simulink model "ten_to_64"  (R2012b)
settings: Solver=FixedStepDiscrete  SolverMode=SingleTasking  StartTime=0.0  StopTime=20000  FixedStep=1  RelTol=1e-3
libraries: xbsIndex_r4 x424, xps_library x1
(part 1 of 3)
settings Model: Creator=paulp  LastModifiedBy=paulp
settings DataIOCC: LimitDataPoints=off
settings OptimizationCC: SimCompilerOptimization=On

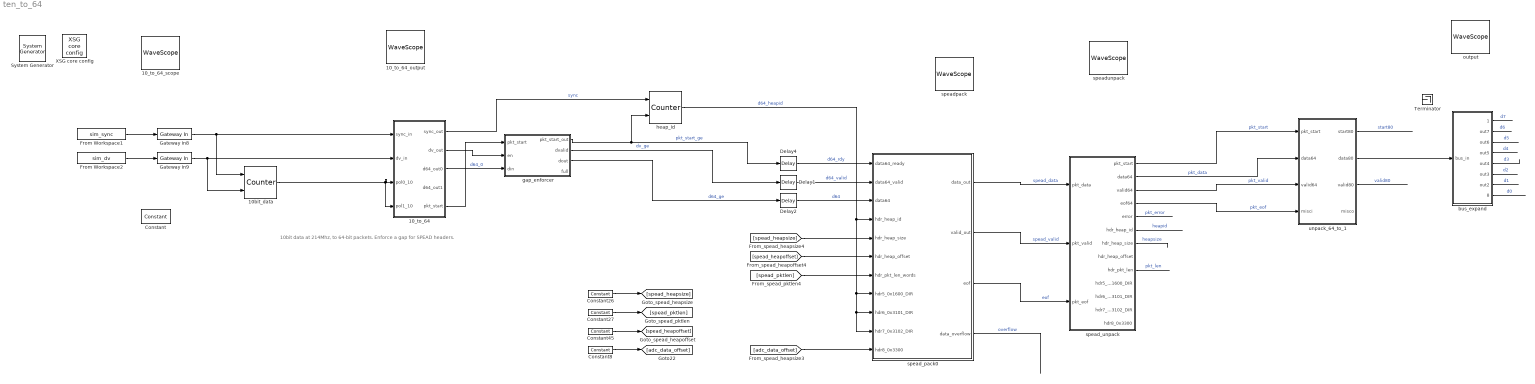
== system ten_to_64 ==
  note: 10bit data at 214Mhz, to 64-bit packets.
      | Enforce a gap for SPEAD headers.
  " System Generator" : xbsIndex_r4/ System Generator  Tag=genX  xilinxfamily=virtex6  part=xc6vsx475t  speed=-1  package=ff1759  synthesis_tool=XST  clock_wrapper=Clock Enables  directory=./netlist  proj_type=Project Navigator  Synth_file=XST Defaults  Impl_file=ISE Defaults  testbench=off  simulink_period=1  sysclk_period=10  dcm_input_clock_period=10  incr_netlist=off  trim_vbits=Everywhere in SubSystem  dbl_ovrd=According to Block Masks  core_generation=According to Block Masks  run_coregen=off  deprecated_control=off  eval_field=0  block_type=sysgen
  10_to_64 : Subsystem
  10_to_64_output : xbsIndex_r4/WaveScope  block_type=wavescope
  10_to_64_scope : xbsIndex_r4/WaveScope  block_type=wavescope
  10bit_data : xbsIndex_r4/Counter  cnt_type=Free Running  cnt_to=Inf  operation=Up  start_count=0  cnt_by_val=1  arith_type=Unsigned  n_bits=10  bin_pt=0  load_pin=off  rst=on  en=on  explicit_period=on  period=1  dbl_ovrd=off  use_behavioral_HDL=off  implementation=Fabric  block_type=counter
  Constant : xbsIndex_r4/Constant  const=1  gui_display_data_type=Boolean  arith_type=Boolean  n_bits=16  bin_pt=14  preci_type=Single  exp_width=8  frac_width=24  explicit_period=on  period=1  equ=P=C  opselect=C  inp2=PCIN>>17  opr=+  inp1=P  carry=CIN  dbl_ovrd=off  block_type=constant
  Constant26 : xbsIndex_r4/Constant  const=4096*10/8  gui_display_data_type=Fixed-point  arith_type=Unsigned  n_bits=48  bin_pt=0  preci_type=Single  exp_width=8  frac_width=24  explicit_period=on  period=1  equ=P=C  opselect=C  inp2=PCIN>>17  opr=+  inp1=P  carry=CIN  dbl_ovrd=off  block_type=constant
  Constant27 : xbsIndex_r4/Constant  const=(4096*10/8)/8  gui_display_data_type=Fixed-point  arith_type=Unsigned  n_bits=48  bin_pt=0  preci_type=Single  exp_width=8  frac_width=24  explicit_period=on  period=1  equ=P=C  opselect=C  inp2=PCIN>>17  opr=+  inp1=P  carry=CIN  dbl_ovrd=off  block_type=constant
  Constant45 : xbsIndex_r4/Constant  const=0  gui_display_data_type=Fixed-point  arith_type=Unsigned  n_bits=48  bin_pt=0  preci_type=Single  exp_width=8  frac_width=24  explicit_period=on  period=1  equ=P=C  opselect=C  inp2=PCIN>>17  opr=+  inp1=P  carry=CIN  dbl_ovrd=off  block_type=constant
  Constant8 : xbsIndex_r4/Constant  const=0  gui_display_data_type=Fixed-point  arith_type=Unsigned  n_bits=48  bin_pt=0  preci_type=Single  exp_width=8  frac_width=24  explicit_period=on  period=1  equ=P=C  opselect=C  inp2=PCIN>>17  opr=+  inp1=P  carry=CIN  dbl_ovrd=off  block_type=constant
  Delay1 : xbsIndex_r4/Delay  rst=off  infoeditControl=Selection of Reset will increase slice count due to use of real FFs and instead of SRLs  en=off  latency=1  dbl_ovrd=off  reg_retiming=off  block_type=delay
  Delay2 : xbsIndex_r4/Delay  rst=off  infoeditControl=Selection of Reset will increase slice count due to use of real FFs and instead of SRLs  en=off  latency=1  dbl_ovrd=off  reg_retiming=off  block_type=delay
  Delay4 : xbsIndex_r4/Delay  rst=off  infoeditControl=Selection of Reset will increase slice count due to use of real FFs and instead of SRLs  en=off  latency=1  dbl_ovrd=off  reg_retiming=off  block_type=delay
  From Workspace1 : FromWorkspace  VariableName=sim_sync  SampleTime=1  Interpolate=off  OutputAfterFinalValue=Setting to zero
  From Workspace2 : FromWorkspace  VariableName=sim_dv  SampleTime=1  Interpolate=off  OutputAfterFinalValue=Setting to zero
  Gateway In8 : xbsIndex_r4/Gateway In  gui_display_data_type=Boolean  arith_type=Boolean  n_bits=10  bin_pt=9  preci_type=Single  exp_width=8  frac_width=24  quantization="Round  (unbiased: +/- Inf)"  overflow=Saturate  period=1  dbl_ovrd=off  timing_constraint=None  locs_specified=off  LOCs={}  UseAsADC=off  ADCChannel='1'  inherit_from_input=off  hdl_port=on  block_type=gatewayin
  Gateway In9 : xbsIndex_r4/Gateway In  gui_display_data_type=Boolean  arith_type=Boolean  n_bits=10  bin_pt=9  preci_type=Single  exp_width=8  frac_width=24  quantization="Round  (unbiased: +/- Inf)"  overflow=Saturate  period=1  dbl_ovrd=off  timing_constraint=None  locs_specified=off  LOCs={}  UseAsADC=off  ADCChannel='1'  inherit_from_input=off  hdl_port=on  block_type=gatewayin
  Terminator : Terminator
  XSG core config : xps_library/XSG core config  Tag=xps:xsg  hw_sys=ROACH2:sx475t  clk_src=sys_clk  ROACH_clk_src=sys_clk  ROACH2_clk_src=sys_clk  MKDIG_clk_src=sys_clk  clk_rate=229  sample_period=1  synthesis_tool=XST
  bus_expand : Subsystem  AncestorBlock=casper_library_flow_control/bus_expand  mask(bus_expand){mode=divisions of equal size, outputNum=8, outputWidth=10, outputBinaryPt=0, outputArithmeticType=0, show_format=on, outputToWorkspace=off, variablePrefix=out, outputToModelAsWell=on}
      mask prompts: outputNum "Number of outputs:"; outputWidth "Output width:"; outputBinaryPt "Output binary point position:"; outputArithmeticType "Output arithmetic type (ufix=0, fix=1, bool=2):"; show_format "Print format string?"; outputToWorkspace "Output to workspace?"; variablePrefix "Variable name prefix:"; outputToModelAsWell "Output to model as well?"
      mask help:
      | Expands a 'bus' made using a bus_create or Xilinx
      | concat block.
      | The input will be divided into the specified number
      | of outputs with the specified arithmetic types.
      | Divisions are made from most significant bit.
      mask init:
      | bus_expand_init(gcb,...
      |     'mode', mode, ...
      |     'outputNum', outputNum, ...
      |     'outputWidth', outputWidth, ...
      |     'outputBinaryPt', outputBinaryPt, ...
      |     'outputArithmeticType', outputArithmeticType, ...
      |     'show_format', show_format, ...
      |     'outputToWorkspace', outputToWorkspace, ...
      |     'variablePrefix', variablePrefix, ...
      |     'outputToModelAsWell', outputToModelAsWell);
      settings: AttributesFormatString=8 outputs: uf10.0,uf10.0,uf10.0,uf10.0,uf10.0,uf10.0,uf10.0,uf10.0,
      mask TypeOptions mode: divisions of equal size | divisions of arbitrary size
      mask Callback mode: bus_expand_callback();
      mask Callback outputWidth: bus_expand_callback();
      mask Callback outputToWorkspace: bus_expand_callback();
  gap_enforcer : Subsystem  mask{block_size=2^(8-1), gap_size=15}
      mask prompts: block_size "data block size"; gap_size "gap size"
  heap_id : xbsIndex_r4/Counter  cnt_type=Free Running  cnt_to=Inf  operation=Up  start_count=0  cnt_by_val=1  arith_type=Unsigned  n_bits=48  bin_pt=0  load_pin=off  rst=on  en=on  explicit_period=on  period=1  dbl_ovrd=off  use_behavioral_HDL=off  implementation=Fabric  block_type=counter
  output : xbsIndex_r4/WaveScope  block_type=wavescope
  spead_pack0 : Subsystem  Tag=casper:spead_pack  AncestorBlock=casper_library_communications/spead_pack  mask(pkt_pack_mask){max_pkt_len_bits=10, header_ids=0x1600, 0x3101, 0x3102, header_ind_ids=0x3300, spead_msw=64, spead_lsw=48, spead_version=4, bytes_per_word=8}
      mask prompts: max_pkt_len_bits "Max pkt length, 2^? 64-bit words"; header_ids "SPEAD direct address IDs (decimal)"; header_ind_ids "SPEAD indirect address IDs (decimal)"; spead_msw "SPEAD Flavour (MSw)"; spead_lsw "SPEAD Flavour (LSw)"; spead_version "SPEAD version"; bytes_per_word "Word size, in bytes"
      mask help:
      | This block generates SPEAD-compliant packets from a datastream.
      |
      | Packets are created with a fixed header followed by a number of 64-bit items.
      |
      | Requires a 64-bit data stream.
      |
      | The data_ready signal is one cycle BEFORE valid data! Does not have to be with a valid signal either.
      mask init:
      | if floor(log2(bytes_per_word)) ~= log2(bytes_per_word)
      |     error('Bytes per word should be a power of two.');
      | end
      | 
      | spead_pack_init(gcb)
  spead_unpack : Subsystem  Tag=casper:spead_unpack  AncestorBlock=casper_library_communications/spead_unpack  mask(spead_unpack_mask){max_pkt_len_bits=10, header_ids=0x1600, 0x3101, 0x3102, header_ind_ids=0x3300, spead_msw=64, spead_lsw=48, spead_version=4, combine_errors=on}
      mask prompts: max_pkt_len_bits "Max pkt length, 2^? 64-bit words"; header_ids "SPEAD direct header IDs (decimal)"; header_ind_ids "SPEAD indirect address IDs (decimal)"; spead_msw "SPEAD Flavour (MSw)"; spead_lsw "SPEAD Flavour (LSw)"; spead_version "SPEAD version"; combine_errors "Combine error flags"
      mask help: This block receives a 64-bit-word stream that contains a SPEAD stream. It checks the SPEAD headers are being correctly received. It presents the user with all headers on the first valid cycle of data along with a flag to indicate a header or packet-length error.
      mask init:
      | spead_unpack_init(gcb)
  speadpack : xbsIndex_r4/WaveScope  block_type=wavescope
  speadunpack : xbsIndex_r4/WaveScope  block_type=wavescope
  unpack_64_to_1 : Subsystem
  wires:
  From Workspace1/1 -> Gateway In8/1
  From Workspace2/1 -> Gateway In9/1
  Gateway In8/1 -> 10bit_data/1, 10_to_64/1(sync_in)
  10bit_data/1 -> 10_to_64/3(pol0_10), 10_to_64/4(pol1_10)
  Gateway In9/1 -> 10bit_data/2, 10_to_64/2(dv_in)
  unpack_64_to_1/1(start80) -> ?  "start80"
  unpack_64_to_1/3(valid80) -> ?  "valid80"
  unpack_64_to_1/2(data80) -> bus_expand/1(bus_in)
  bus_expand/1(msb_out8) -> ?  "d7"
  bus_expand/2(out7) -> ?  "d6"
  bus_expand/3(out6) -> ?  "d5"
  bus_expand/4(out5) -> ?  "d4"
  bus_expand/5(out4) -> ?  "d3"
  bus_expand/6(out3) -> ?  "d2"
  bus_expand/7(out2) -> ?  "d1"
  bus_expand/8(lsb_out1) -> ?  "d0"
  Constant26/1 -> [spead_heapsize]
  Constant27/1 -> [spead_pktlen]
  Constant45/1 -> [spead_heapoffset]
  Constant8/1 -> [adc_data_offset]
  [spead_heapsize] -> spead_pack0/5(hdr_heap_size)
  [spead_heapoffset] -> spead_pack0/6(hdr_heap_offset)
  [spead_pktlen] -> spead_pack0/7(hdr_pkt_len_words)
  [adc_data_offset] -> spead_pack0/11(hdr8_0x3300)
  heap_id/1 -> spead_pack0/10(hdr7_0x3102_DIR), spead_pack0/9(hdr6_0x3101_DIR), spead_pack0/8(hdr5_0x1600_DIR), spead_pack0/4(hdr_heap_id)  "d64_heapid"
  spead_pack0/1(data_out) -> spead_unpack/1(pkt_data)  "spead_data"
  spead_pack0/2(valid_out) -> spead_unpack/2(pkt_valid)  "spead_valid"
  spead_pack0/3(eof) -> spead_unpack/3(pkt_eof)  "eof"
  spead_pack0/4(data_overflow) -> ?  "overflow"
  10_to_64/1(sync_out) -> heap_id/1  "sync"
  10_to_64/3(d64_out0) -> gap_enforcer/3(din)  "d64_0"
  10_to_64/2(dv_out) -> gap_enforcer/2(en)
  spead_unpack/4(eof64) -> unpack_64_to_1/4(misci)  "pkt_eof"
  spead_unpack/6(hdr_heap_id) -> ?  "heapid"
  spead_unpack/5(error) -> ?  "pkt_error"
  spead_unpack/7(hdr_heap_size) -> ?  "heapsize"
  spead_unpack/9(hdr_pkt_len) -> ?  "pkt_len"
  10_to_64/5(pkt_start) -> gap_enforcer/1(pkt_start)
  spead_unpack/1(pkt_start) -> unpack_64_to_1/1(pkt_start)  "pkt_start"
  spead_unpack/2(data64) -> unpack_64_to_1/2(data64)  "pkt_data"
  spead_unpack/3(valid64) -> unpack_64_to_1/3(valid64)  "pkt_valid"
  Delay4/1 -> spead_pack0/1(data64_ready)  "d64_rdy"
  Delay1/1 -> spead_pack0/2(data64_valid)  "d64_valid"
  Delay2/1 -> spead_pack0/3(data64)  "d64"
  gap_enforcer/1(pkt_start_out) -> heap_id/2, Delay4/1  "pkt_start_ge"
  gap_enforcer/2(dvalid) -> Delay1/1  "dv_ge"
  gap_enforcer/3(dout) -> Delay2/1  "d64_ge"

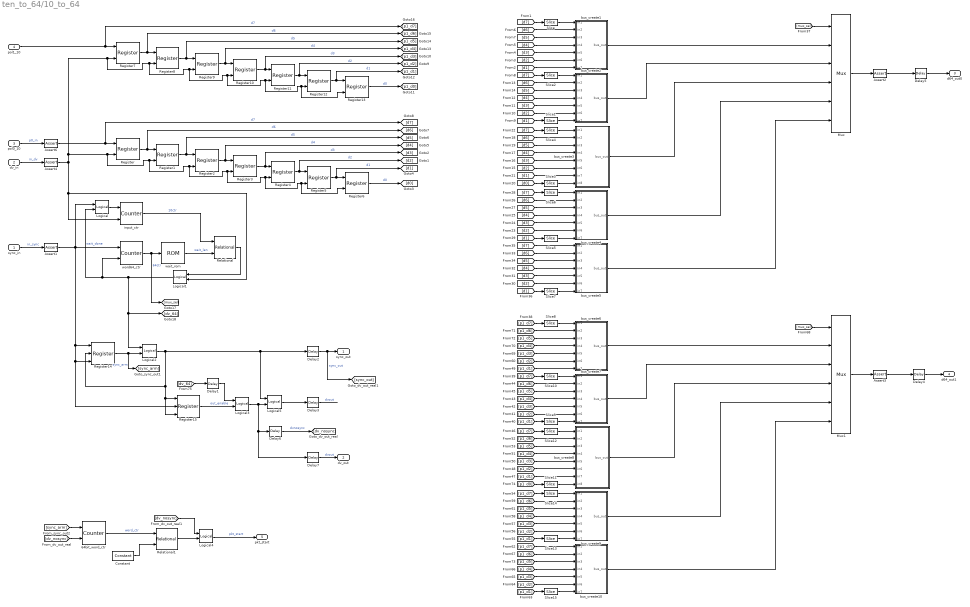
== system ten_to_64/10_to_64 ==
  sync_in : Inport
  dv_in : Inport  Port=2
  pol0_10 : Inport  Port=3
  pol1_10 : Inport  Port=4
  64bit_word_ctr : xbsIndex_r4/Counter  cnt_type=Count Limited  cnt_to=639  operation=Up  start_count=0  cnt_by_val=1  arith_type=Unsigned  n_bits=10  bin_pt=0  load_pin=off  rst=on  en=on  explicit_period=on  period=1  dbl_ovrd=off  use_behavioral_HDL=off  implementation=Fabric  block_type=counter
  Assert1 : xbsIndex_r4/Assert  assert_type=on  type_source=Explicitly  gui_display_data_type=Boolean  arith_type=Boolean  n_bits=80  bin_pt=0  preci_type=Single  exp_width=8  frac_width=24  assert_rate=off  rate_source=Explicitly  period=1  output_port=on  block_type=assert
      settings: block_version=10.1.3
  Assert2 : xbsIndex_r4/Assert  assert_type=on  type_source=Explicitly  gui_display_data_type=Fixed-point  arith_type=Unsigned  n_bits=64  bin_pt=0  preci_type=Single  exp_width=8  frac_width=24  assert_rate=off  rate_source=Explicitly  period=1  output_port=on  block_type=assert
      settings: block_version=10.1.3
  Assert3 : xbsIndex_r4/Assert  assert_type=on  type_source=Explicitly  gui_display_data_type=Fixed-point  arith_type=Unsigned  n_bits=64  bin_pt=0  preci_type=Single  exp_width=8  frac_width=24  assert_rate=off  rate_source=Explicitly  period=1  output_port=on  block_type=assert
      settings: block_version=10.1.3
  Assert4 : xbsIndex_r4/Assert  assert_type=on  type_source=Explicitly  gui_display_data_type=Boolean  arith_type=Boolean  n_bits=80  bin_pt=0  preci_type=Single  exp_width=8  frac_width=24  assert_rate=off  rate_source=Explicitly  period=1  output_port=on  block_type=assert
      settings: block_version=10.1.3
  Assert6 : xbsIndex_r4/Assert  assert_type=on  type_source=Explicitly  gui_display_data_type=Fixed-point  arith_type=Unsigned  n_bits=10  bin_pt=0  preci_type=Single  exp_width=8  frac_width=24  assert_rate=off  rate_source=Explicitly  period=1  output_port=on  block_type=assert
      settings: block_version=10.1.3
  Constant : xbsIndex_r4/Constant  const=0  gui_display_data_type=Fixed-point  arith_type=Unsigned  n_bits=10  bin_pt=0  preci_type=Single  exp_width=8  frac_width=24  explicit_period=on  period=1  equ=P=C  opselect=C  inp2=PCIN>>17  opr=+  inp1=P  carry=CIN  dbl_ovrd=off  block_type=constant
  Delay1 : xbsIndex_r4/Delay  rst=off  infoeditControl=Selection of Reset will increase slice count due to use of real FFs and instead of SRLs  en=off  latency=1  dbl_ovrd=off  reg_retiming=off  block_type=delay
  Delay{2..5,7} (5 alike) : xbsIndex_r4/Delay  rst=off  infoeditControl=Selection of Reset will increase slice count due to use of real FFs and instead of SRLs  en=off  latency=2  dbl_ovrd=off  reg_retiming=off  block_type=delay
  Delay6 : xbsIndex_r4/Delay  rst=off  infoeditControl=Selection of Reset will increase slice count due to use of real FFs and instead of SRLs  en=off  latency=1  dbl_ovrd=off  reg_retiming=off  block_type=delay
  Logical : xbsIndex_r4/Logical  logical_function=OR  inputs=2  en=off  latency=0  precision=Full  arith_type=Unsigned  n_bits=16  bin_pt=0  align_bp=on  dbl_ovrd=off  block_type=logical
  Logical{1..4} (4 alike) : xbsIndex_r4/Logical  logical_function=AND  inputs=2  en=off  latency=0  precision=Full  arith_type=Unsigned  n_bits=16  bin_pt=0  align_bp=on  dbl_ovrd=off  block_type=logical
  Logical5 : xbsIndex_r4/Logical  logical_function=OR  inputs=2  en=off  latency=0  precision=Full  arith_type=Unsigned  n_bits=16  bin_pt=0  align_bp=on  dbl_ovrd=off  block_type=logical
  Mux : xbsIndex_r4/Mux  inputs=5  en=off  latency=1  precision=Full  arith_type=Unsigned  n_bits=16  bin_pt=14  quantization=Truncate  overflow=Wrap  dbl_ovrd=off  block_type=mux
  Mux1 : xbsIndex_r4/Mux  inputs=5  en=off  latency=1  precision=Full  arith_type=Unsigned  n_bits=16  bin_pt=14  quantization=Truncate  overflow=Wrap  dbl_ovrd=off  block_type=mux
  Register{,1..13} (14 alike) : xbsIndex_r4/Register  init=0  rst=off  en=on  dbl_ovrd=off  block_type=register
  Register14 : xbsIndex_r4/Register  init=0  rst=on  en=on  dbl_ovrd=off  block_type=register
  Register15 : xbsIndex_r4/Register  init=0  rst=on  en=on  dbl_ovrd=off  block_type=register
  Relational : xbsIndex_r4/Relational  mode=a=b  en=off  latency=0  dbl_ovrd=off  block_type=relational
  Relational1 : xbsIndex_r4/Relational  mode=a=b  en=off  latency=0  dbl_ovrd=off  block_type=relational
  Slice : xbsIndex_r4/Slice  nbits=4  boolean_output=off  mode=Lower Bit Location + Width  bit1=0  base1=MSB of Input  bit0=0  base0=LSB of Input  dbl_ovrd=off  block_type=slice
  Slice1 : xbsIndex_r4/Slice  nbits=6  boolean_output=off  mode=Upper Bit Location + Width  bit1=0  base1=MSB of Input  bit0=0  base0=LSB of Input  dbl_ovrd=off  block_type=slice
  Slice10 : xbsIndex_r4/Slice  nbits=8  boolean_output=off  mode=Lower Bit Location + Width  bit1=0  base1=MSB of Input  bit0=0  base0=LSB of Input  dbl_ovrd=off  block_type=slice
  Slice11 : xbsIndex_r4/Slice  nbits=2  boolean_output=off  mode=Upper Bit Location + Width  bit1=0  base1=MSB of Input  bit0=0  base0=LSB of Input  dbl_ovrd=off  block_type=slice
  Slice12 : xbsIndex_r4/Slice  nbits=2  boolean_output=off  mode=Lower Bit Location + Width  bit1=0  base1=MSB of Input  bit0=0  base0=LSB of Input  dbl_ovrd=off  block_type=slice
  Slice13 : xbsIndex_r4/Slice  nbits=8  boolean_output=off  mode=Upper Bit Location + Width  bit1=0  base1=MSB of Input  bit0=0  base0=LSB of Input  dbl_ovrd=off  block_type=slice
  Slice14 : xbsIndex_r4/Slice  nbits=6  boolean_output=off  mode=Lower Bit Location + Width  bit1=0  base1=MSB of Input  bit0=0  base0=LSB of Input  dbl_ovrd=off  block_type=slice
  Slice15 : xbsIndex_r4/Slice  nbits=4  boolean_output=off  mode=Upper Bit Location + Width  bit1=0  base1=MSB of Input  bit0=0  base0=LSB of Input  dbl_ovrd=off  block_type=slice
  Slice2 : xbsIndex_r4/Slice  nbits=8  boolean_output=off  mode=Lower Bit Location + Width  bit1=0  base1=MSB of Input  bit0=0  base0=LSB of Input  dbl_ovrd=off  block_type=slice
  Slice3 : xbsIndex_r4/Slice  nbits=2  boolean_output=off  mode=Upper Bit Location + Width  bit1=0  base1=MSB of Input  bit0=0  base0=LSB of Input  dbl_ovrd=off  block_type=slice
  Slice4 : xbsIndex_r4/Slice  nbits=2  boolean_output=off  mode=Lower Bit Location + Width  bit1=0  base1=MSB of Input  bit0=0  base0=LSB of Input  dbl_ovrd=off  block_type=slice
  Slice5 : xbsIndex_r4/Slice  nbits=8  boolean_output=off  mode=Upper Bit Location + Width  bit1=0  base1=MSB of Input  bit0=0  base0=LSB of Input  dbl_ovrd=off  block_type=slice
  Slice6 : xbsIndex_r4/Slice  nbits=6  boolean_output=off  mode=Lower Bit Location + Width  bit1=0  base1=MSB of Input  bit0=0  base0=LSB of Input  dbl_ovrd=off  block_type=slice
  Slice7 : xbsIndex_r4/Slice  nbits=4  boolean_output=off  mode=Upper Bit Location + Width  bit1=0  base1=MSB of Input  bit0=0  base0=LSB of Input  dbl_ovrd=off  block_type=slice
  Slice8 : xbsIndex_r4/Slice  nbits=4  boolean_output=off  mode=Lower Bit Location + Width  bit1=0  base1=MSB of Input  bit0=0  base0=LSB of Input  dbl_ovrd=off  block_type=slice
  Slice9 : xbsIndex_r4/Slice  nbits=6  boolean_output=off  mode=Upper Bit Location + Width  bit1=0  base1=MSB of Input  bit0=0  base0=LSB of Input  dbl_ovrd=off  block_type=slice
  bus_create1 : Subsystem  AncestorBlock=casper_library_flow_control/bus_create  mask(bus_create){inputNum=7}
      mask prompts: inputNum "Number of inputs:"
      mask init:
      | bus_create_init(gcb,...
      |     'inputNum', inputNum);
  bus_create10 : Subsystem  AncestorBlock=casper_library_flow_control/bus_create  mask(bus_create){inputNum=7}
      mask prompts: inputNum "Number of inputs:"
      mask init:
      | bus_create_init(gcb,...
      |     'inputNum', inputNum);
  bus_create2 : Subsystem  AncestorBlock=casper_library_flow_control/bus_create  mask(bus_create){inputNum=7}
      mask prompts: inputNum "Number of inputs:"
      mask init:
      | bus_create_init(gcb,...
      |     'inputNum', inputNum);
  bus_create3 : Subsystem  AncestorBlock=casper_library_flow_control/bus_create  mask(bus_create){inputNum=8}
      mask prompts: inputNum "Number of inputs:"
      mask init:
      | bus_create_init(gcb,...
      |     'inputNum', inputNum);
  bus_create4 : Subsystem  AncestorBlock=casper_library_flow_control/bus_create  mask(bus_create){inputNum=7}
      mask prompts: inputNum "Number of inputs:"
      mask init:
      | bus_create_init(gcb,...
      |     'inputNum', inputNum);
  bus_create5 : Subsystem  AncestorBlock=casper_library_flow_control/bus_create  mask(bus_create){inputNum=7}
      mask prompts: inputNum "Number of inputs:"
      mask init:
      | bus_create_init(gcb,...
      |     'inputNum', inputNum);
  bus_create6 : Subsystem  AncestorBlock=casper_library_flow_control/bus_create  mask(bus_create){inputNum=7}
      mask prompts: inputNum "Number of inputs:"
      mask init:
      | bus_create_init(gcb,...
      |     'inputNum', inputNum);
  bus_create7 : Subsystem  AncestorBlock=casper_library_flow_control/bus_create  mask(bus_create){inputNum=7}
      mask prompts: inputNum "Number of inputs:"
      mask init:
      | bus_create_init(gcb,...
      |     'inputNum', inputNum);
  bus_create8 : Subsystem  AncestorBlock=casper_library_flow_control/bus_create  mask(bus_create){inputNum=8}
      mask prompts: inputNum "Number of inputs:"
      mask init:
      | bus_create_init(gcb,...
      |     'inputNum', inputNum);
  bus_create9 : Subsystem  AncestorBlock=casper_library_flow_control/bus_create  mask(bus_create){inputNum=7}
      mask prompts: inputNum "Number of inputs:"
      mask init:
      | bus_create_init(gcb,...
      |     'inputNum', inputNum);
  input_ctr : xbsIndex_r4/Counter  cnt_type=Free Running  cnt_to=Inf  operation=Up  start_count=0  cnt_by_val=1  arith_type=Unsigned  n_bits=4  bin_pt=0  load_pin=off  rst=on  en=on  explicit_period=on  period=1  dbl_ovrd=off  use_behavioral_HDL=off  implementation=Fabric  block_type=counter
  wait_rom : xbsIndex_r4/ROM  depth=5  initVector=[6 5 6 5 5]  distributed_mem=Distributed memory  rst=off  init_reg=0  en=off  latency=0  gui_display_data_type=Fixed-point  arith_type=Unsigned  n_bits=4  bin_pt=0  preci_type=Single  exp_width=8  frac_width=24  dbl_ovrd=off  optimize=Area  use_rpm=on  block_type=sprom
  word64_ctr : xbsIndex_r4/Counter  cnt_type=Count Limited  cnt_to=4  operation=Up  start_count=0  cnt_by_val=1  arith_type=Unsigned  n_bits=3  bin_pt=0  load_pin=off  rst=on  en=on  explicit_period=on  period=1  dbl_ovrd=off  use_behavioral_HDL=off  implementation=Fabric  block_type=counter
  sync_out : Outport
  dv_out : Outport  Port=2
  d64_out0 : Outport  Port=3
  d64_out1 : Outport  Port=4
  pkt_start : Outport  Port=5
  wires:
  sync_in/1 -> Assert1/1  "in_sync"
  pol0_10/1 -> Assert6/1  "p0_in"
  dv_in/1 -> Assert4/1  "in_dv"
  Register/1 -> [d6], Register1/1  "d6"
  Assert6/1 -> [d7], Register/1  "d7"
  Register5/1 -> [d1], Register6/1  "d1"
  Register4/1 -> [d2], Register5/1  "d2"
  Register3/1 -> [d3], Register4/1  "d3"
  Register2/1 -> [d4], Register3/1  "d4"
  Register1/1 -> [d5], Register2/1  "d5"
  [d7] -> Slice/1
  Slice/1 -> bus_create1/1(in1)
  [d6] -> bus_create1/2(in2)
  [d5] -> bus_create1/3(in3)
  [d4] -> bus_create1/4(in4)
  [d1] -> bus_create1/7(in7)
  [d3] -> bus_create1/5(in5)
  [d2] -> bus_create1/6(in6)
  bus_create1/1(bus_out) -> Mux/2
  [d7] -> Slice2/1
  Slice2/1 -> bus_create2/1(in1)
  [d6] -> bus_create2/2(in2)
  [d5] -> bus_create2/3(in3)
  [d4] -> bus_create2/4(in4)
  [d1] -> Slice1/1
  [d3] -> bus_create2/5(in5)
  [d2] -> bus_create2/6(in6)
  Slice1/1 -> bus_create2/7(in7)
  bus_create2/1(bus_out) -> Mux/3
  [d0] -> Slice3/1
  Slice3/1 -> bus_create3/8(in8)
  [d7] -> Slice4/1
  Slice4/1 -> bus_create3/1(in1)
  [d3] -> bus_create3/5(in5)
  [d2] -> bus_create3/6(in6)
  [d4] -> bus_create3/4(in4)
  [d6] -> bus_create3/2(in2)
  [d5] -> bus_create3/3(in3)
  [d1] -> bus_create3/7(in7)
  [d7] -> Slice6/1
  Slice6/1 -> bus_create4/1(in1)
  [d6] -> bus_create4/2(in2)
  [d5] -> bus_create4/3(in3)
  [d4] -> bus_create4/4(in4)
  [d1] -> Slice5/1
  [d3] -> bus_create4/5(in5)
  [d2] -> bus_create4/6(in6)
  Slice5/1 -> bus_create4/7(in7)
  [d7] -> bus_create5/1(in1)
  [d6] -> bus_create5/2(in2)
  [d5] -> bus_create5/3(in3)
  [d4] -> bus_create5/4(in4)
  [d1] -> Slice7/1
  [d3] -> bus_create5/5(in5)
  [d2] -> bus_create5/6(in6)
  Slice7/1 -> bus_create5/7(in7)
  [mux_sel] -> Mux/1
  bus_create3/1(bus_out) -> Mux/4
  bus_create4/1(bus_out) -> Mux/5
  bus_create5/1(bus_out) -> Mux/6
  Register6/1 -> [d0]  "d0"
  Assert1/1 -> Logical/1, Register15/2, Register14/3, Register14/1, word64_ctr/1
  word64_ctr/1 -> [mux_sel], wait_rom/1  "64ctr"
  wait_rom/1 -> Relational/2  "wait_len"
  input_ctr/1 -> Relational/1  "10ctr"
  Relational/1 -> Logical1/1
  Logical1/1 -> [dv_64], Logical2/1, word64_ctr/2, Logical/2  "wait_done"
  Logical/1 -> input_ctr/1
  Register7/1 -> Register8/1, [p1_d6]  "d6"
  pol1_10/1 -> Register7/1, [p1_d7]  "d7"
  Register12/1 -> Register13/1, [p1_d1]  "d1"
  Register11/1 -> Register12/1, [p1_d2]  "d2"
  Register10/1 -> Register11/1, [p1_d3]  "d3"
  Register9/1 -> Register10/1, [p1_d4]  "d4"
  Register8/1 -> Register9/1, [p1_d5]  "d5"
  Register13/1 -> [p1_d0]  "d0"
  Assert4/1 -> Logical1/2, input_ctr/2, Register8/2, Register9/2, Register10/2, Register11/2, Register12/2, Register13/2, Register7/2, Register6/2, Register5/2, Register4/2, Register3/2, Register2/2, Register1/2, Register/2
  [p1_d7] -> Slice8/1
  Slice8/1 -> bus_create6/1(in1)
  [p1_d6] -> bus_create6/2(in2)
  [p1_d5] -> bus_create6/3(in3)
  [p1_d4] -> bus_create6/4(in4)
  [p1_d1] -> bus_create6/7(in7)
  [p1_d3] -> bus_create6/5(in5)
  [p1_d2] -> bus_create6/6(in6)
  bus_create6/1(bus_out) -> Mux1/2
  [p1_d7] -> Slice10/1
  Slice10/1 -> bus_create7/1(in1)
  [p1_d6] -> bus_create7/2(in2)
  [p1_d5] -> bus_create7/3(in3)
  [p1_d4] -> bus_create7/4(in4)
  [p1_d1] -> Slice9/1
  [p1_d3] -> bus_create7/5(in5)
  [p1_d2] -> bus_create7/6(in6)
  Slice9/1 -> bus_create7/7(in7)
  bus_create7/1(bus_out) -> Mux1/3
  [p1_d0] -> Slice11/1
  Slice11/1 -> bus_create8/8(in8)
  [p1_d7] -> Slice12/1
  Slice12/1 -> bus_create8/1(in1)
  [p1_d3] -> bus_create8/5(in5)
  [p1_d2] -> bus_create8/6(in6)
  [p1_d4] -> bus_create8/4(in4)
  [p1_d6] -> bus_create8/2(in2)
  [p1_d5] -> bus_create8/3(in3)
  [p1_d1] -> bus_create8/7(in7)
  [p1_d7] -> Slice14/1
  Slice14/1 -> bus_create9/1(in1)
  [p1_d6] -> bus_create9/2(in2)
  [p1_d5] -> bus_create9/3(in3)
  [p1_d4] -> bus_create9/4(in4)
  [p1_d1] -> Slice13/1
  [p1_d3] -> bus_create9/5(in5)
  [p1_d2] -> bus_create9/6(in6)
  Slice13/1 -> bus_create9/7(in7)
  [p1_d7] -> bus_create10/1(in1)
  [p1_d6] -> bus_create10/2(in2)
  [p1_d5] -> bus_create10/3(in3)
  [p1_d4] -> bus_create10/4(in4)
  [p1_d1] -> Slice15/1
  [p1_d3] -> bus_create10/5(in5)
  [p1_d2] -> bus_create10/6(in6)
  Slice15/1 -> bus_create10/7(in7)
  [mux_sel] -> Mux1/1
  bus_create8/1(bus_out) -> Mux1/4
  bus_create9/1(bus_out) -> Mux1/5
  bus_create10/1(bus_out) -> Mux1/6
  Mux/1 -> Assert2/1
  Mux1/1 -> Assert3/1
  Assert2/1 -> Delay5/1
  Assert3/1 -> Delay4/1
  Register14/1 -> [sync_arm], Logical2/2  "sync_arm"
  Logical2/1 -> Delay2/1, Logical5/1, Register15/3, Register15/1, Register14/2
  Register15/1 -> Logical3/2  "out_enable"
  [dv_64] -> Delay1/1
  Logical5/1 -> Delay3/1
  [sync_arm] -> 64bit_word_ctr/1
  [dv_nosync] -> 64bit_word_ctr/2
  Logical3/1 -> Delay7/1, Delay6/1, Logical5/2
  Delay1/1 -> Logical3/1
  Delay2/1 -> [sync_out], sync_out/1  "sync_out"
  Delay3/1 -> ?  "dvout"
  Delay4/1 -> d64_out1/1
  Delay5/1 -> d64_out0/1
  Logical4/1 -> pkt_start/1  "pkt_start"
  64bit_word_ctr/1 -> Relational1/1  "word_ctr"
  Delay6/1 -> [dv_nosync]  "dvnosync"
  Constant/1 -> Relational1/2
  Relational1/1 -> Logical4/2
  [dv_nosync] -> Logical4/1
  Delay7/1 -> dv_out/1  "dvout"

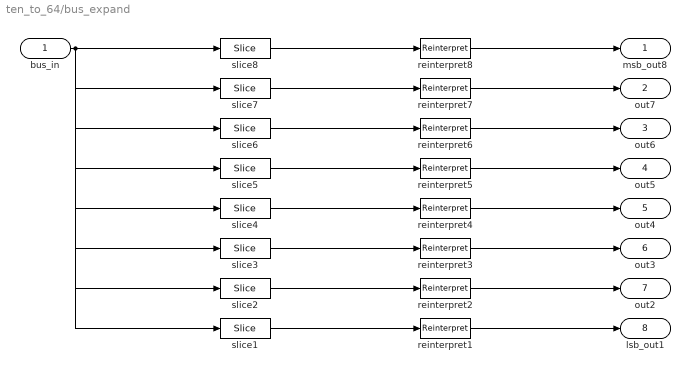
== system ten_to_64/bus_expand ==
  bus_in : Inport
  reinterpret{1..8} (8 alike) : xbsIndex_r4/Reinterpret  force_arith_type=on  arith_type=Unsigned  force_bin_pt=on  bin_pt=0  block_type=reinterpret
  slice1 : xbsIndex_r4/Slice  nbits=10  boolean_output=off  mode=Upper Bit Location + Width  bit1=-70  base1=MSB of Input  bit0=0  base0=LSB of Input  dbl_ovrd=off  block_type=slice
  slice2 : xbsIndex_r4/Slice  nbits=10  boolean_output=off  mode=Upper Bit Location + Width  bit1=-60  base1=MSB of Input  bit0=0  base0=LSB of Input  dbl_ovrd=off  block_type=slice
  slice3 : xbsIndex_r4/Slice  nbits=10  boolean_output=off  mode=Upper Bit Location + Width  bit1=-50  base1=MSB of Input  bit0=0  base0=LSB of Input  dbl_ovrd=off  block_type=slice
  slice4 : xbsIndex_r4/Slice  nbits=10  boolean_output=off  mode=Upper Bit Location + Width  bit1=-40  base1=MSB of Input  bit0=0  base0=LSB of Input  dbl_ovrd=off  block_type=slice
  slice5 : xbsIndex_r4/Slice  nbits=10  boolean_output=off  mode=Upper Bit Location + Width  bit1=-30  base1=MSB of Input  bit0=0  base0=LSB of Input  dbl_ovrd=off  block_type=slice
  slice6 : xbsIndex_r4/Slice  nbits=10  boolean_output=off  mode=Upper Bit Location + Width  bit1=-20  base1=MSB of Input  bit0=0  base0=LSB of Input  dbl_ovrd=off  block_type=slice
  slice7 : xbsIndex_r4/Slice  nbits=10  boolean_output=off  mode=Upper Bit Location + Width  bit1=-10  base1=MSB of Input  bit0=0  base0=LSB of Input  dbl_ovrd=off  block_type=slice
  slice8 : xbsIndex_r4/Slice  nbits=10  boolean_output=off  mode=Upper Bit Location + Width  bit1=0  base1=MSB of Input  bit0=0  base0=LSB of Input  dbl_ovrd=off  block_type=slice
  msb_out8 : Outport
  out7 : Outport  Port=2
  out6 : Outport  Port=3
  out5 : Outport  Port=4
  out4 : Outport  Port=5
  out3 : Outport  Port=6
  out2 : Outport  Port=7
  lsb_out1 : Outport  Port=8
  wires:
  bus_in/1 -> slice8/1, slice7/1, slice6/1, slice5/1, slice4/1, slice3/1, slice2/1, slice1/1
  slice8/1 -> reinterpret8/1
  reinterpret8/1 -> msb_out8/1
  slice7/1 -> reinterpret7/1
  reinterpret7/1 -> out7/1
  slice6/1 -> reinterpret6/1
  reinterpret6/1 -> out6/1
  slice5/1 -> reinterpret5/1
  reinterpret5/1 -> out5/1
  slice4/1 -> reinterpret4/1
  reinterpret4/1 -> out4/1
  slice3/1 -> reinterpret3/1
  reinterpret3/1 -> out3/1
  slice2/1 -> reinterpret2/1
  reinterpret2/1 -> out2/1
  slice1/1 -> reinterpret1/1
  reinterpret1/1 -> lsb_out1/1

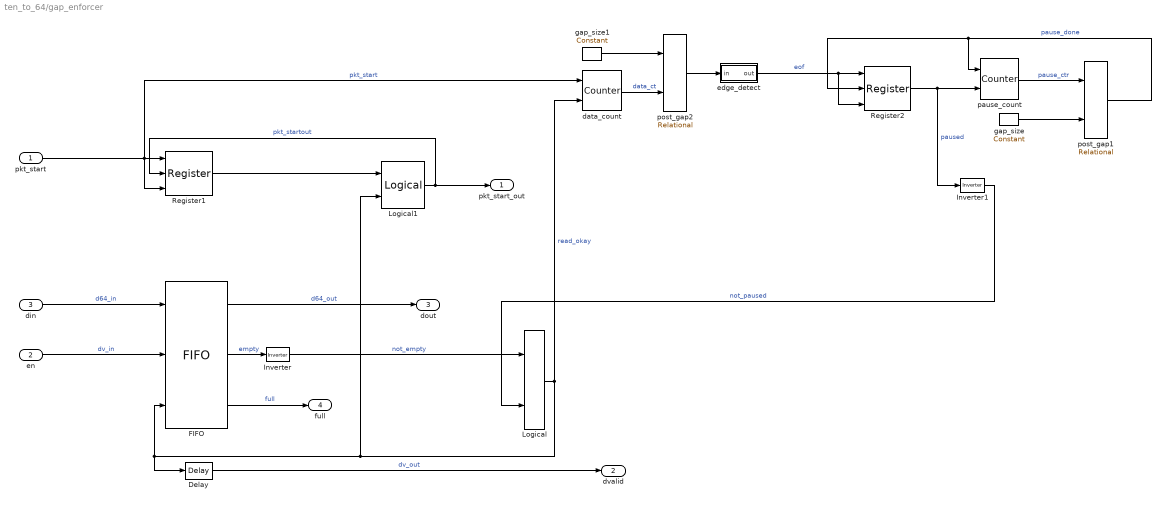
== system ten_to_64/gap_enforcer ==
  pkt_start : Inport
  en : Inport  Port=2
  din : Inport  Port=3
  Delay : xbsIndex_r4/Delay  rst=off  infoeditControl=Selection of Reset will increase slice count due to use of real FFs and instead of SRLs  en=off  latency=1  dbl_ovrd=off  reg_retiming=off  block_type=delay
  FIFO : xbsIndex_r4/FIFO  mem_type=Distributed RAM  performance_options=Standard_FIFO  infoedit1=Available only for V4, V5, V6, V7, K7, A7 and Zynq devices.  embedded_registers=off  depth=32  percent_nbits=2  rst=off  en=off  use_dcount=off  use_percent_full_port=off  use_almost_empty=off  almost_empty_thresh=2  use_almost_full=off  almost_full_thresh=14  dbl_ovrd=off  explicit_period=off  block_type=fifo
  Inverter : xbsIndex_r4/Inverter  en=off  latency=0  dbl_ovrd=off  block_type=inv
  Inverter1 : xbsIndex_r4/Inverter  en=off  latency=0  dbl_ovrd=off  block_type=inv
  Logical : xbsIndex_r4/Logical  logical_function=AND  inputs=2  en=off  latency=0  precision=Full  arith_type=Unsigned  n_bits=16  bin_pt=0  align_bp=on  dbl_ovrd=off  block_type=logical
  Logical1 : xbsIndex_r4/Logical  logical_function=AND  inputs=2  en=off  latency=0  precision=Full  arith_type=Unsigned  n_bits=16  bin_pt=0  align_bp=on  dbl_ovrd=off  block_type=logical
  Register1 : xbsIndex_r4/Register  init=0  rst=on  en=on  dbl_ovrd=off  block_type=register
  Register2 : xbsIndex_r4/Register  init=0  rst=on  en=on  dbl_ovrd=off  block_type=register
  data_count : xbsIndex_r4/Counter  cnt_type=Free Running  cnt_to=15  operation=Up  start_count=0  cnt_by_val=1  arith_type=Unsigned  n_bits=10  bin_pt=0  load_pin=off  rst=on  en=on  explicit_period=on  period=1  dbl_ovrd=off  use_behavioral_HDL=off  implementation=Fabric  block_type=counter
  edge_detect : Subsystem  AncestorBlock=casper_library_misc/edge_detect  mask(edge_detect){edge=Rising, polarity=Active High, x_in=[0 0.08 0.08 0.16 0.16 0.24 0.24 0.32 0.32 0.4], y_in=[-1 -1  1  1  1  1  1  1  1  1], x_out=[0.6 0.68 0.68 0.76 0.76 0.84 0.84 0.92 0.92 1], y_out=[-1 -1  1  1 -1 -1 -1 -1 -1 -1]}
      mask prompts: edge "Edge Type"; polarity "Output Polarity"; x_in "Input X Positions"; y_in "Input Y Positions"; x_out "Output X Positions"; y_out "Output Y Positions"
      mask help: Output is active for one-cycle after each edge of the specified type (i.e. rising, falling or both).
      mask init:
      | edge_detect_init(gcb,...
      |     'edge',edge,...
      |     'polarity',polarity,...
      |     'x_in',x_in,...
      |     'x_out',x_out,...
      |     'y_in',y_in,...
      |     'y_out',y_out);
      | 
      | x_in_num=str2num(getfield(getfield(get_param(gcb,'UserData'),'parameters'),'x_in'));
      | x_out_num=str2num(getfield(getfield(get_param(gcb,'UserData'),'parameters'),'x_out'));
      | y_in_num=str2num(getfield(getfield(get_param(gcb,'UserData'),'parameters'),'y_in'));
      | y_out_num=str2num(getfield(getfield(get_param(gcb,'UserData'),'parameters'),'y_out'));
      settings: AttributesFormatString=|
      | rising edges
      | active high
      mask Help: Output is active for one-cycle after each edge of the specified type (i.e. rising, falling, or both).  Latency is zero.
      mask TypeOptions edge: Rising | Falling | Both
      mask TypeOptions polarity: Active High | Active Low
      mask Display:
      | plot(x_in_num,0.5+y_in_num*0.2);
      | plot(x_out_num,0.5+y_out_num*0.2);
  gap_size : xbsIndex_r4/Constant  const=15  gui_display_data_type=Fixed-point  arith_type=Unsigned  n_bits=ceil(log2(15))  bin_pt=0  preci_type=Single  exp_width=8  frac_width=24  explicit_period=on  period=1  equ=P=C  opselect=C  inp2=PCIN>>17  opr=+  inp1=P  carry=CIN  dbl_ovrd=off  block_type=constant
  gap_size1 : xbsIndex_r4/Constant  const=640  gui_display_data_type=Fixed-point  arith_type=Unsigned  n_bits=10  bin_pt=0  preci_type=Single  exp_width=8  frac_width=24  explicit_period=on  period=1  equ=P=C  opselect=C  inp2=PCIN>>17  opr=+  inp1=P  carry=CIN  dbl_ovrd=off  block_type=constant
  pause_count : xbsIndex_r4/Counter  cnt_type=Count Limited  cnt_to=15  operation=Up  start_count=0  cnt_by_val=1  arith_type=Unsigned  n_bits=ceil(log2(15))  bin_pt=0  load_pin=off  rst=on  en=on  explicit_period=on  period=1  dbl_ovrd=off  use_behavioral_HDL=off  implementation=Fabric  block_type=counter
  post_gap1 : xbsIndex_r4/Relational  mode=a=b  en=off  latency=0  dbl_ovrd=off  block_type=relational
  post_gap2 : xbsIndex_r4/Relational  mode=a=b  en=off  latency=0  dbl_ovrd=off  block_type=relational
  pkt_start_out : Outport
  dvalid : Outport  Port=2
  dout : Outport  Port=3
  full : Outport  Port=4
  wires:
  Logical/1 -> Logical1/2, FIFO/3, Delay/1, data_count/2  "read_okay"
  FIFO/2 -> Inverter/1  "empty"
  FIFO/3 -> full/1  "full"
  Inverter/1 -> Logical/1  "not_empty"
  din/1 -> FIFO/1  "d64_in"
  Delay/1 -> dvalid/1  "dv_out"
  en/1 -> FIFO/2  "dv_in"
  data_count/1 -> post_gap2/2  "data_ct"
  gap_size1/1 -> post_gap2/1
  post_gap2/1 -> edge_detect/1(in)
  edge_detect/1(out) -> Register2/3, Register2/1  "eof"
  Register2/1 -> Inverter1/1, pause_count/2  "paused"
  pkt_start/1 -> Register1/3, data_count/1, Register1/1  "pkt_start"
  FIFO/1 -> dout/1  "d64_out"
  gap_size/1 -> post_gap1/2
  pause_count/1 -> post_gap1/1  "pause_ctr"
  post_gap1/1 -> pause_count/1, Register2/2  "pause_done"
  Inverter1/1 -> Logical/2  "not_paused"
  Register1/1 -> Logical1/1
  Logical1/1 -> Register1/2, pkt_start_out/1  "pkt_startout"
